simulink model "WirelessChannelSimulation"  (R2021a)
settings: Solver=VariableStepAuto  StartTime=0.0  StopTime=200  RelTol=1e-3
undefined symbols (not defined in the file): entity, m, n, WirelessListener
libraries: simulink x1
settings Model: Creator=The MathWorks, Inc.  LastModifiedBy=mluser
settings SolverCC: AlgebraicLoopSolver=TrustRegion
settings DebuggingCC: SFMachineParentedDataDiag=warning

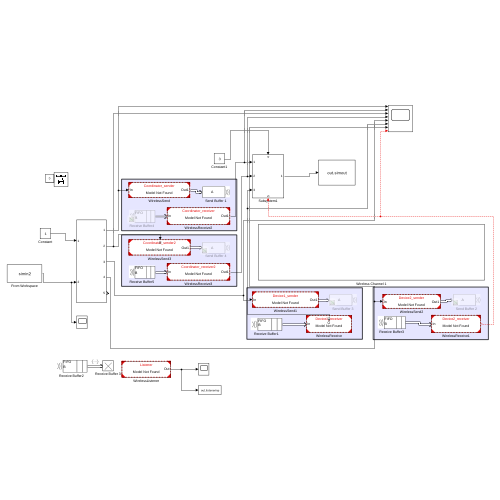
[thumbnail: Simulink's stored preview of the top-level diagram]
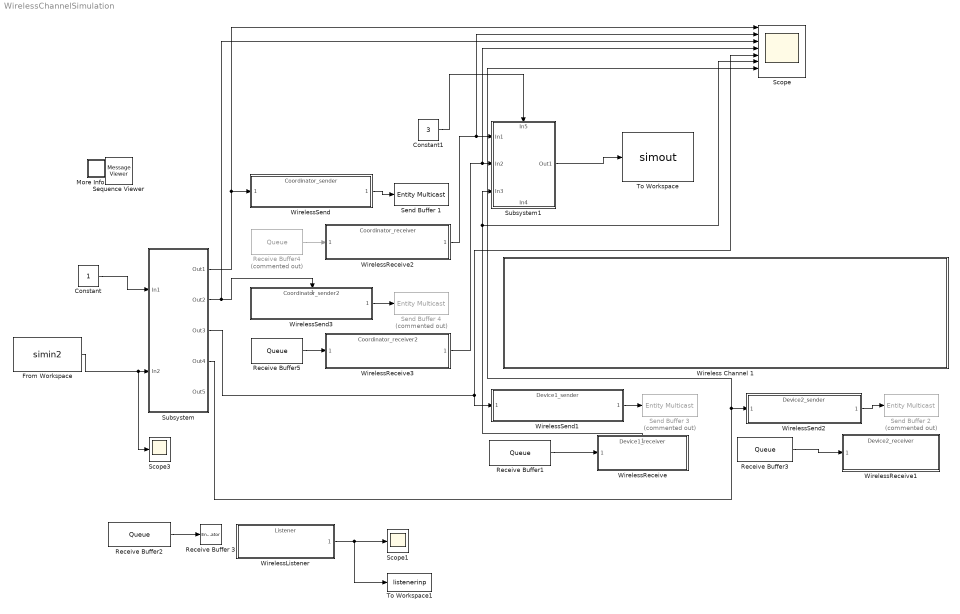
== system WirelessChannelSimulation ==
  Constant : Constant
  Constant1 : Constant  Value=3
  From Workspace : FromWorkspace  LoadFcn=|  VariableName=simin2
      | OWPAN_SSID = '1111111111112200';
      |     
      | %     a = timer('ExecutionMode','fixedRate','Period',10,'TimerFcn',@myfun,'TasksToExecute',10);
      | %     start(a);
      |     
      |     beacon = Create_beacon(OWPAN_SSID);
      |     
      |           
      |     beacon = double(beacon);
      |     time = 1:1:length(beacon);
      |     
      |     % Binary information as stream of bits (binary signal 0 or 1)
      |     disp('Beacon Frame generated and Sending -Binary information: ');
      |     disp(beacon);
      |     
      |     load_system('Coordinator_sender');
      |     load_system('Device1_sender');
      |     load_system('Device2_sender');
      |     
      |     set_param('WirelessChannelSimulation', 'StopTime',  num2str(length(beacon)));
      |     set_param('Coordinator_sender/From Workspace','commented','off');
      |     set_param('WirelessChannelSimulation/Send Buffer 1','commented','off');
      |     set_param('Device1_sender/From Workspace','commented','on');
      |     set_param('WirelessChannelSimulation/Send Buffer 3','commented','on');
      |     set_param('Device2_sender/From Workspace','commented','on');
      |     set_param('WirelessChannelSimulation/Send Buffer 2','commented','on');
      |     
      |     %Call simulink model
      |     simin = [time.',beacon.'];
      |     sim('WirelessChannelSimulation.slx');
      | 
      | %     wait(a);
      | %     disp('Beacon Sent');
  More Info : Subsystem
      settings: OpenFcn=showExample('simulink/MessageCommunicationPacketLossChannelFailureExample')
      mask Display: disp('?')
  Receive Buffer 3 : EntityTerminator  InputPortMessageModes=m  EntryAction=WirelessListener.onOneMessage(entity);
  Receive Buffer{1..3,5} (4 alike) : Queue  OutputPortMessageModes=m  Capacity=16  EntityArrivalSource=Multicast  MulticastTag=B
  Receive Buffer4 : Queue  Commented=on  OutputPortMessageModes=m  Capacity=16  EntityArrivalSource=Multicast  MulticastTag=B
  Scope : Scope  NumInputPorts=8
  Scope1 : Scope
  Scope3 : Scope
  Send Buffer 1 : EntityMulticast  InputPortMessageModes=m
  Send Buffer 2 : EntityMulticast  Commented=on  InputPortMessageModes=m
  Send Buffer 3 : EntityMulticast  Commented=on  InputPortMessageModes=m
  Send Buffer 4 : EntityMulticast  Commented=on  InputPortMessageModes=m
  Sequence Viewer : MessageViewer  History=1000  SavedRootId=#
  Subsystem : Subsystem
  Subsystem1 : Subsystem
      settings: PortSchema="{\"entries\":[{\"content\":{\"sides\":[{\"content\":{\"connectorIds\":[\"In1\",\"In2\",\"In3\"]},\"type\":\"ConnectorPlacement.EquallySpacedRectSide\",\"uuid\":\"355ae0f0-6a2b-4df0-a695-f8a4027a74b4\"},{\"content\":{\"connectorIds\":[\"Out1\"],\"side\":\"RIGHT\"},\"type\":\"ConnectorPlacement.EquallySpacedRectSide\",\"uuid\":\"192bb8ad-cad8-44a0-b230-a407f18e16db\"},{\"content\":{\"connectorIds\":[\"In4\"],\"side\":\"TOP\"},\"type\":\"ConnectorPlacement.EquallySpacedRectSide\",\"uuid\":\"b2d4a3b0-752a-4ec8-9eea-1dadc6e34edf\"},{\"content\":{\"connectorIds\":[\"In5\"],\"side\":\"BOTTOM\"},\"type\":\"ConnectorPlacement.EquallySpacedRectSide\",\"uuid\":\"0af7b35c-3126-4142-8602-8e08258d01b1\"}]},\"type\":\"ConnectorPlacement.EquallySpacedConnector\",\"uuid\":\"5693e41e-d0e8-41e4-aefc-b4df0bc35316\"}],\"packageUris\":[\"http://schema.mathworks.com/mf0/Connector/R2020b\"],\"version\":\"1.0\"}"
  To Workspace : ToWorkspace  VariableName=simout  SaveFormat=Timeseries  SampleTime=-1
  To Workspace1 : ToWorkspace  VariableName=listenerinp  SaveFormat=Timeseries  SampleTime=-1
      settings: MaxDataPoints=1
  Wireless Channel 1 : Subsystem
  WirelessListener : ModelReference  ModelNameDialog=Listener.slx  SimulationMode=Normal  ScheduleRates=on  ModelReferenceVersion=3.0
  WirelessReceive : ModelReference  InputPortMessageModes=m  ModelNameDialog=Device1_receiver.slx  SimulationMode=Normal  ModelReferenceVersion=3.29
      settings: PortSchema="{\"entries\":[{\"content\":{\"sides\":[{\"content\":{\"connectorIds\":[\"In1\"]},\"type\":\"ConnectorPlacement.EquallySpacedRectSide\",\"uuid\":\"a99da9cd-0138-497f-8456-d2ca8a1e68af\"},{\"content\":{\"connectorIds\":[],\"side\":\"RIGHT\"},\"type\":\"ConnectorPlacement.EquallySpacedRectSide\",\"uuid\":\"a0aee5c5-57dc-49d3-94ec-52271de65030\"},{\"content\":{\"connectorIds\":[\"Out1\"],\"side\":\"TOP\"},\"type\":\"ConnectorPlacement.EquallySpacedRectSide\",\"uuid\":\"339029b6-9323-49a3-8c30-a34a15e757d1\"}]},\"type\":\"ConnectorPlacement.EquallySpacedConnector\",\"uuid\":\"c5391053-1bac-4aad-b490-90d373c3a3bc\"}],\"packageUris\":[\"http://schema.mathworks.com/mf0/Connector/R2020b\"],\"version\":\"1.0\"}"
  WirelessReceive1 : ModelReference  InputPortMessageModes=m  ModelNameDialog=Device2_receiver.slx  SimulationMode=Normal  ModelReferenceVersion=3.12
  WirelessReceive2 : ModelReference  InputPortMessageModes=m  ModelNameDialog=Coordinator_receiver.slx  SimulationMode=Normal  ModelReferenceVersion=3.18
  WirelessReceive3 : ModelReference  InputPortMessageModes=m  ModelNameDialog=Coordinator_receiver2.slx  SimulationMode=Normal  ModelReferenceVersion=3.19
  WirelessSend : ModelReference  OutputPortMessageModes=m  ModelNameDialog=Coordinator_sender.slx  SimulationMode=Normal  ModelReferenceVersion=3.96
  WirelessSend1 : ModelReference  OutputPortMessageModes=m  ModelNameDialog=Device1_sender.slx  SimulationMode=Normal  ModelReferenceVersion=3.37
  WirelessSend2 : ModelReference  OutputPortMessageModes=m  ModelNameDialog=Device2_sender.slx  SimulationMode=Normal  ModelReferenceVersion=3.33
  WirelessSend3 : ModelReference  OutputPortMessageModes=m  ModelNameDialog=Coordinator_sender2.slx  SimulationMode=Normal  ModelReferenceVersion=3.42
      settings: PortSchema="{\"entries\":[{\"content\":{\"sides\":[{\"content\":{\"connectorIds\":[]},\"type\":\"ConnectorPlacement.EquallySpacedRectSide\",\"uuid\":\"a99da9cd-0138-497f-8456-d2ca8a1e68af\"},{\"content\":{\"connectorIds\":[\"Out1\"],\"side\":\"RIGHT\"},\"type\":\"ConnectorPlacement.EquallySpacedRectSide\",\"uuid\":\"a0aee5c5-57dc-49d3-94ec-52271de65030\"},{\"content\":{\"connectorIds\":[\"In1\"],\"side\":\"TOP\"},\"type\":\"ConnectorPlacement.EquallySpacedRectSide\",\"uuid\":\"339029b6-9323-49a3-8c30-a34a15e757d1\"}]},\"type\":\"ConnectorPlacement.EquallySpacedConnector\",\"uuid\":\"c5391053-1bac-4aad-b490-90d373c3a3bc\"}],\"packageUris\":[\"http://schema.mathworks.com/mf0/Connector/R2020b\"],\"version\":\"1.0\"}"
  wires:
  Receive Buffer1/1 -> WirelessReceive/1
  Receive Buffer2/1 -> Receive Buffer 3/1
  WirelessSend/1 -> Send Buffer 1/1
  Receive Buffer3/1 -> WirelessReceive1/1
  Receive Buffer4/1 -> WirelessReceive2/1
  WirelessSend1/1 -> Send Buffer 3/1
  WirelessSend2/1 -> Send Buffer 2/1
  WirelessSend3/1 -> Send Buffer 4/1
  Receive Buffer5/1 -> WirelessReceive3/1
  WirelessReceive3/1 -> Scope/4, Subsystem1/2(In2)
  WirelessReceive/1 -> Scope/6, Subsystem1/3(In3)
  Subsystem1/1(Out1) -> To Workspace/1
  From Workspace/1 -> Scope3/1, Subsystem/2(In2)
  Constant/1 -> Subsystem/1(In1)
  Subsystem/1(Out1) -> Scope/1, WirelessSend/1
  Subsystem/2(Out2) -> Scope/3, WirelessSend3/1
  Subsystem/3(Out3) -> WirelessSend1/1, Scope/5
  Subsystem/4(Out4) -> Scope/7, WirelessSend2/1
  ? -> Scope/8, Subsystem1/5(In4)
  Constant1/1 -> Subsystem1/4(In5)
  WirelessReceive2/1 -> Scope/2, Subsystem1/1(In1)
  WirelessListener/1 -> To Workspace1/1, Scope1/1

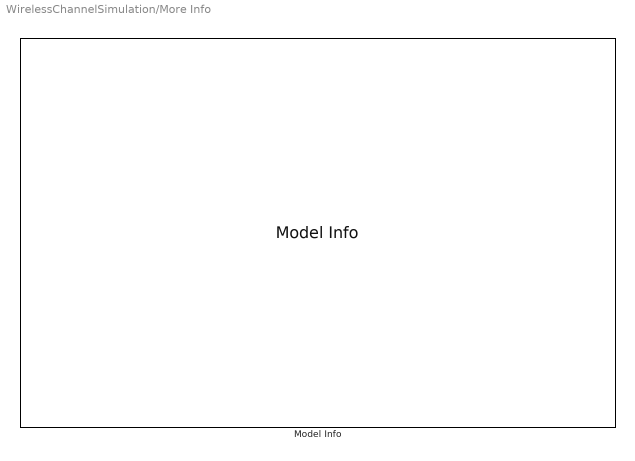
== system WirelessChannelSimulation/More Info ==
  Model Info : simulink/Model-Wide Utilities/Model Info  Frame=on  DisplayStringWithTags=|  HorizontalTextAlignment=Left  LeftAlignmentValue=0.02
      | Model Description:
      | -------------------
      | This example shows how to use the Message Delay block to model a variable
      | speed conveyor belt between two airport terminals. The passengers step on
      | the conveyor belt following a Poisson distribution. Since passengers are
      | discrete entities, they are naturally modeled by Simulink(R) messages,
      | which are created by the Entity Generator block. When a passenger, i.e.,
      | a Simulink(R) message, is sent to the Message Delay block, the block
      | will hold it until it arrives at the other end of the conveyor belt. The
      | length of the delay time is automatically calculated by Simulink(R) based
      | on the ETA (estimated time of arrival), which is calculated by the
      | Stateflow(R) Chart. The operation of the conveyor belt depends on the
      | load and its transfer characteristics.

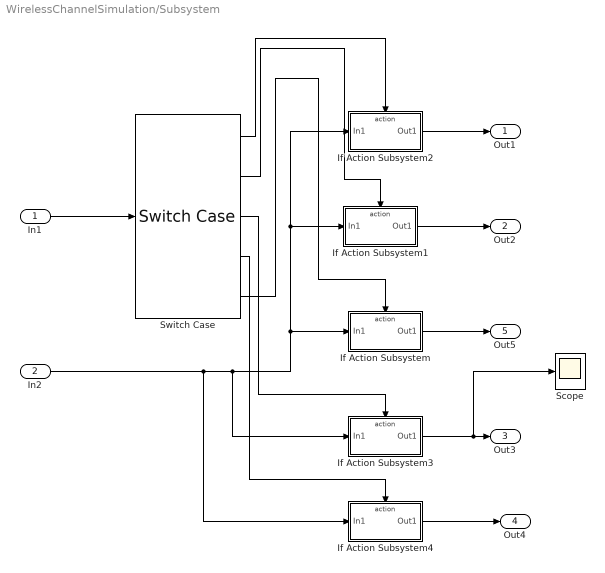
== system WirelessChannelSimulation/Subsystem ==
  In1 : Inport
  In2 : Inport  Port=2
  If Action Subsystem : Subsystem  TreatAsAtomicUnit=on
  If Action Subsystem1 : Subsystem  TreatAsAtomicUnit=on
  If Action Subsystem2 : Subsystem  TreatAsAtomicUnit=on
  If Action Subsystem3 : Subsystem  TreatAsAtomicUnit=on
  If Action Subsystem4 : Subsystem  TreatAsAtomicUnit=on
  Scope : Scope
  Switch Case : SwitchCase  CaseConditions={1, 2,3,4}
  Out1 : Outport
  Out2 : Outport  Port=2
  Out3 : Outport  Port=3
  Out4 : Outport  Port=4
  Out5 : Outport  Port=5
  wires:
  Switch Case/1 -> If Action Subsystem2/Action
  Switch Case/2 -> If Action Subsystem1/Action
  In1/1 -> Switch Case/1
  In2/1 -> If Action Subsystem4/1(In1), If Action Subsystem3/1(In1), If Action Subsystem1/1(In1), If Action Subsystem2/1(In1), If Action Subsystem/1(In1)
  Switch Case/5 -> If Action Subsystem/Action
  If Action Subsystem1/1(Out1) -> Out2/1
  If Action Subsystem/1(Out1) -> Out5/1
  If Action Subsystem2/1(Out1) -> Out1/1
  Switch Case/3 -> If Action Subsystem3/Action
  If Action Subsystem3/1(Out1) -> Scope/1, Out3/1
  Switch Case/4 -> If Action Subsystem4/Action
  If Action Subsystem4/1(Out1) -> Out4/1

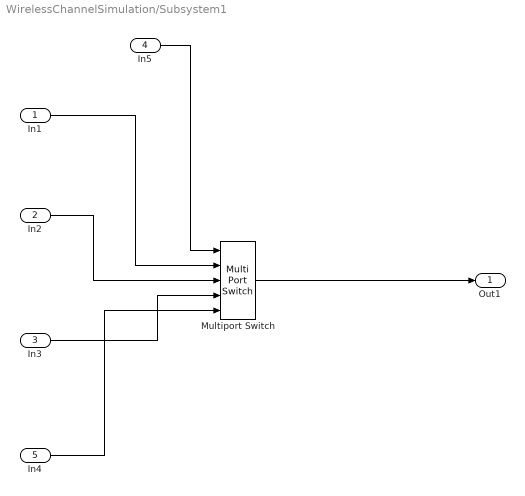
== system WirelessChannelSimulation/Subsystem1 ==
  In1 : Inport
  In2 : Inport  Port=2
  In3 : Inport  Port=3
  In5 : Inport  Port=4
  In4 : Inport  Port=5
  Multiport Switch : MultiPortSwitch  Inputs=4
  Out1 : Outport
  wires:
  In1/1 -> Multiport Switch/2
  In2/1 -> Multiport Switch/3
  In3/1 -> Multiport Switch/4
  In4/1 -> Multiport Switch/5
  Multiport Switch/1 -> Out1/1
  In5/1 -> Multiport Switch/1

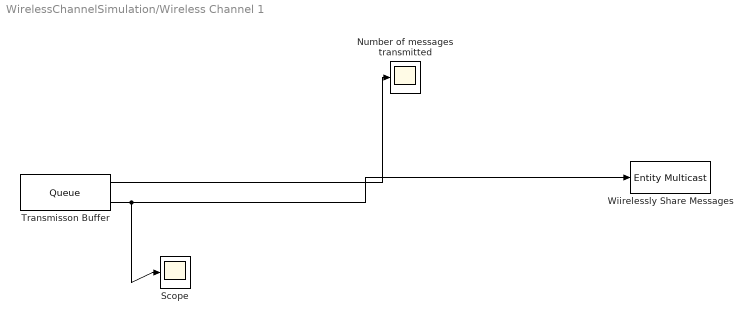
== system WirelessChannelSimulation/Wireless Channel 1 ==
  Number of messages transmitted : Scope
  Scope : Scope
  Transmisson Buffer : Queue  OutputPortMessageModes=n,m  Capacity=100  EntityArrivalSource=Multicast  NumberEntitiesDeparted=on
      settings: OutputPortMap=o0,o5
  Wiirelessly Share Messages : EntityMulticast  InputPortMessageModes=m  MulticastTag=B
  wires:
  Transmisson Buffer/1 -> Number of messages transmitted/1
  Transmisson Buffer/2 -> Scope/1, Wiirelessly Share Messages/1

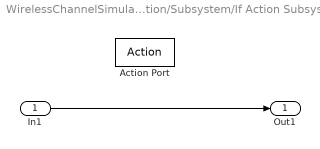
== system WirelessChannelSimulation/Subsystem/If Action Subsystem ==
  In1 : Inport
  Action Port : ActionPort  ActionPortLabel=default:
  Out1 : Outport
  wires:
  In1/1 -> Out1/1

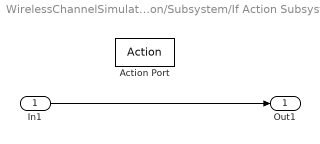
== system WirelessChannelSimulation/Subsystem/If Action Subsystem1 ==
  In1 : Inport
  Action Port : ActionPort  ActionPortLabel=case [ 2 ]:
  Out1 : Outport
  wires:
  In1/1 -> Out1/1

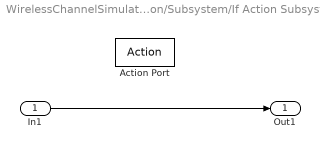
== system WirelessChannelSimulation/Subsystem/If Action Subsystem2 ==
  In1 : Inport
  Action Port : ActionPort  ActionPortLabel=case [ 1 ]:
  Out1 : Outport
  wires:
  In1/1 -> Out1/1

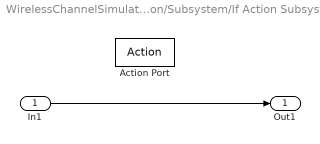
== system WirelessChannelSimulation/Subsystem/If Action Subsystem3 ==
  In1 : Inport
  Action Port : ActionPort  ActionPortLabel=case [ 3 ]:
  Out1 : Outport
  wires:
  In1/1 -> Out1/1

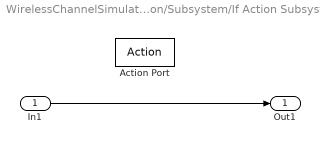
== system WirelessChannelSimulation/Subsystem/If Action Subsystem4 ==
  In1 : Inport
  Action Port : ActionPort  ActionPortLabel=case [ 4 ]:
  Out1 : Outport
  wires:
  In1/1 -> Out1/1
